simulink model "Boost_converter3"  (R2013a)
settings: Solver=ode45  StartTime=0.0  StopTime=10.0  RelTol=1e-3
libraries: powerlib x13
settings Model: Creator=radow  LastModifiedBy=radow

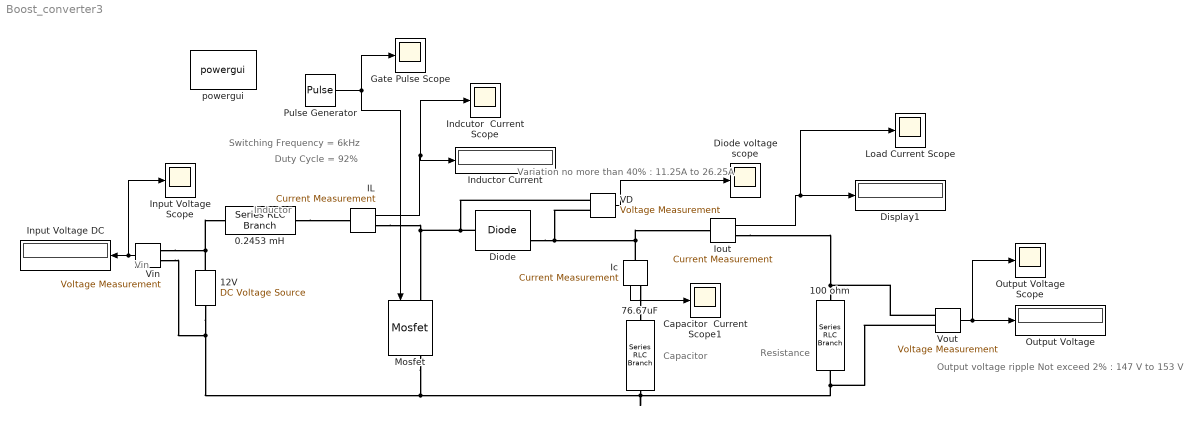
== system Boost_converter3 ==
  note: Vin
  note: Output voltage ripple Not exceed 2% :
      | 147 V to 153 V
  note: Variation no more than 40% :
      | 11.25A to 26.25A
  note: Duty Cycle = 92%
  note: Switching Frequency = 6kHz
  note: Resistance
  note: Capacitor
  note: Inductor
  0.2453 mH : powerlib/Elements/Series RLC Branch  LConnTagsString=__new0  RConnTagsString=__new0  BranchType=L  Resistance=1  Inductance=0.2453e-3  SetiL0=off  InitialCurrent=0  Capacitance=1e-6  Setx0=off  InitialVoltage=0  Measurements=None
  100 ohm : powerlib/Elements/Series RLC Branch  LConnTagsString=__new0  RConnTagsString=__new0  BranchType=R  Resistance=100  Inductance=1e-3  SetiL0=off  InitialCurrent=0  Capacitance=1e-6  Setx0=off  InitialVoltage=0  Measurements=None
  12V : powerlib/Electrical Sources/DC Voltage Source  Amplitude=12  Measurements=None
  76.67uF : powerlib/Elements/Series RLC Branch  LConnTagsString=__new0  RConnTagsString=__new0  BranchType=C  Resistance=1  Inductance=1e-3  SetiL0=off  InitialCurrent=0  Capacitance=76.67e-6  Setx0=off  InitialVoltage=0  Measurements=None
  Capacitor  Current Scope1 : Scope
      settings: ShowLegends=on  TimeRange=20  YMin=-175  YMax=25  SaveName=ScopeData4
  Diode : powerlib/Power Electronics/Diode  Ron=0.00001  Lon=0  Vf=0  IC=0  UseSnubber=off  Rs=0  Cs=0  Measurements=on
  Diode voltage scope : Scope
      settings: ShowLegends=on  TimeRange=20  YMin=-175  YMax=25
  Display1 : Display
  Gate Pulse Scope : Scope
      settings: ShowLegends=on  TimeRange=20  YMin=-175  YMax=25  SaveName=ScopeData2
  IL : powerlib/Measurements/Current Measurement  PhasorSimulation=off  OutputType=Complex  PSBequivalent=0
  Ic : powerlib/Measurements/Current Measurement  PhasorSimulation=off  OutputType=Complex  PSBequivalent=0
  Indcutor  Current Scope : Scope
      settings: ShowLegends=on  TimeRange=20  YMin=-175  YMax=25  SaveName=ScopeData3
  Inductor Current : Display
  Input Voltage DC : Display
  Input Voltage Scope : Scope
      settings: ShowLegends=on  TimeRange=20  YMin=12  YMax=12
  Iout : powerlib/Measurements/Current Measurement  PhasorSimulation=off  OutputType=Complex  PSBequivalent=0
  Load Current Scope : Scope
      settings: ShowLegends=on  TimeRange=20  YMin=-175  YMax=25  SaveName=ScopeData5
  Mosfet : powerlib/Power Electronics/Mosfet  Ron=0.0001  Lon=0  Rd=0.001  Vfd=0  IC=0  Rs=500  Cs=inf  Measurements=on
  Output Voltage : Display
  Output Voltage Scope : Scope
      settings: ShowLegends=on  TimeRange=20  YMin=-175  YMax=25  SaveName=ScopeData6
  Pulse Generator : DiscretePulseGenerator  PulseType=Time based  Period=1/6000  PulseWidth=92
  VD : powerlib/Measurements/Voltage Measurement  PhasorSimulation=off  OutputType=Complex  PSBequivalent=0
  Vin : powerlib/Measurements/Voltage Measurement  PhasorSimulation=off  OutputType=Complex  PSBequivalent=0
  Vout : powerlib/Measurements/Voltage Measurement  PhasorSimulation=off  OutputType=Complex  PSBequivalent=0
  powergui : powerlib/powergui  Priority=1  SimulationMode=Continuous  SolverType=Tustin  SampleTime=50e-6  frequency=60  SPID=off  DisableSnubberDevices=off  DisableRonSwitches=off  DisableVfSwitches=off  SwTol=0  Interpol=off  DisplayEquations=off  frequencyindice=0  Pbase=100e6  ErrMax=1e-4  Iterations=50  UnitsV=kV  UnitsW=MW  FunctionMessages=off  echomessages=off  HookPort=off  EnableUseOfTLC=off  x0status=blocks  RestoreLinks=warning  ResistiveCurrentMeasurement=off  Frange=[0:2:500]  Ylog=off  Xlog=on  ShowGrid=off  save=off  variable=ZData  ZoomFFT=off  StartTime=0.0  cycles=1  DisplayStyle=1  fundamental=60  FreqAxis=off  MaxFrequency=1000  frequencyindicesteady=1  RmsSteady=1  display=off  Ts=0  methode=off
  wires:
  Vout/1 -> Output Voltage Scope/1, Output Voltage/1
  Pulse Generator/1 -> Mosfet/1, Gate Pulse Scope/1
  Vin/1 -> Input Voltage Scope/1, Input Voltage DC/1
  Iout/1 -> Load Current Scope/1, Display1/1
  VD/1 -> Diode voltage scope/1
  IL/1 -> Indcutor  Current Scope/1, Inductor Current/1
  Ic/1 -> Capacitor  Current Scope1/1
  connections:
  Ic/LConn1 -- VD/LConn2 -- Diode/RConn1 -- Iout/LConn1
  100 ohm/RConn1 -- Vout/LConn2 -- 76.67uF/RConn1 -- Vin/LConn2 -- 12V/LConn1 -- Mosfet/RConn1
  Iout/RConn1 -- Vout/LConn1 -- 100 ohm/LConn1
  12V/RConn1 -- Vin/LConn1 -- 0.2453 mH/LConn1
  IL/RConn1 -- VD/LConn1 -- Diode/LConn1 -- Mosfet/LConn1
  Ic/RConn1 -- 76.67uF/LConn1
  0.2453 mH/RConn1 -- IL/LConn1
